simulink model "PIL"  (R2021b)
settings: Solver=FixedStepAuto  StartTime=0.0  StopTime=Inf  RelTol=1e-3
model workspace (MAT data in the model file):
  Ts = 0.001
libraries: arduinomotorcarrierlib x4
settings Model: PacingRate=2  ExtModeTrigDuration=2  Creator=cirie  LastModifiedBy=cirie
settings DataIOCC: SaveOutput=off  SaveTime=off
settings OptimizationCC: EnhancedBackFolding=on  PassReuseOutputArgsAs=Individual arguments  ZeroExternalMemoryAtStartup=off  ZeroInternalMemoryAtStartup=off  MaxStackSize=64  OptimizeBlockOrder=speed  DifferentSizesBufferReuse=on  OptimizationCustomize=off  EfficientTunableParamExpr=on
settings DebuggingCC: ParameterTunabilityLossMsg=error
settings HardwareCC: ProdBitPerPointer=32  ProdBitPerSizeT=32  ProdBitPerPtrDiffT=32  ProdLargestAtomicInteger=Long  ProdLargestAtomicFloat=Double  ProdWordSize=32  ProdHWDeviceType=ARM Compatible->ARM Cortex
settings SFSimCC: MATLABDynamicMemAlloc=off
settings RTWCC: Description=Embedded Coder  SystemTargetFile=ert.tlc  HardwareBoard=Arduino MKR WiFi 1010  TemplateMakefile=ert_default_tmf  Toolchain=Arduino ARM
settings CodeAppCC: ForceParamTrailComments=on  IgnoreCustomStorageClasses=off  OperatorAnnotations=on  SimulinkDataObjDesc=on  SFDataObjDesc=on  InsertBlockDesc=on
settings ERTTargetCC: SupportContinuousTime=on  SupportVariableSizeSignals=on  ExtModeTransport=3  ExtModeStaticAlloc=on  ExtModeStaticAllocSize=8192  ExtModeMexFile=ext_xcp  ExtModeIntrfLevel=Level2 - Open

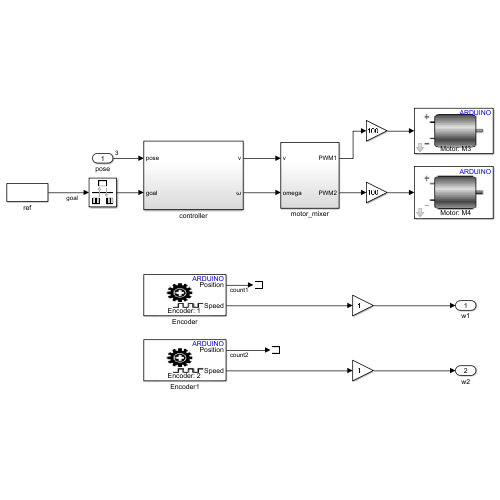
[thumbnail: Simulink's stored preview of the top-level diagram]
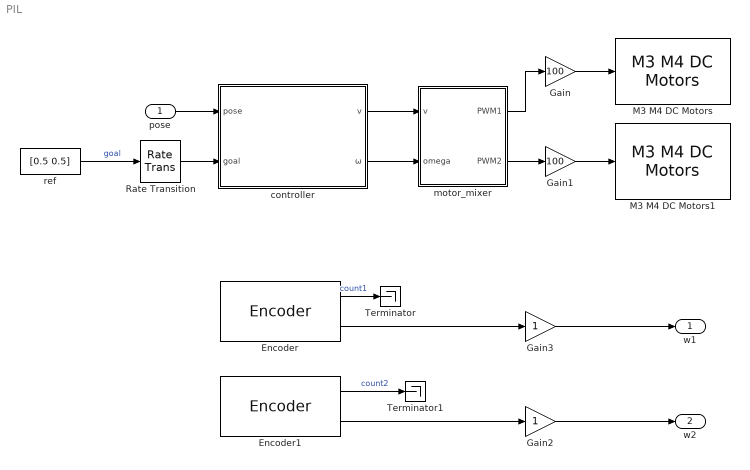
== system PIL ==
  pose : Inport  OutDataTypeStr=single  PortDimensions=3  SampleTime=[0.001,0]
  Encoder : arduinomotorcarrierlib/Encoder  SlaveAddress=uint8( hex2dec( '66' ) )  blockPlatform=ARDUINO  Encoder=1  ShowSpeed=on  ResetOption=on  SampleTime=0.01
      settings: SourceProductBaseCode=ARDUINO
  Encoder1 : arduinomotorcarrierlib/Encoder  SlaveAddress=uint8( hex2dec( '66' ) )  blockPlatform=ARDUINO  Encoder=2  ShowSpeed=on  ResetOption=on  SampleTime=0.01
      settings: SourceProductBaseCode=ARDUINO
  Gain : Gain  Gain=100
  Gain1 : Gain  Gain=100
  Gain2 : Gain
  Gain3 : Gain
  M3 M4 DC Motors : arduinomotorcarrierlib/M3 M4 DC Motors  MotorNumber=M3  forwardPinNumber=3  reversePinNumber=2
      settings: SourceProductBaseCode=ARDUINO
  M3 M4 DC Motors1 : arduinomotorcarrierlib/M3 M4 DC Motors  MotorNumber=M4  forwardPinNumber=4  reversePinNumber=5
      settings: SourceProductBaseCode=ARDUINO
  Rate Transition : RateTransition  OutPortSampleTime=Ts
  Terminator : Terminator
  Terminator1 : Terminator
  controller : Subsystem
  motor_mixer : Subsystem
  ref : Constant  Value=[0.5 0.5]  SampleTime=Ts
  w1 : Outport  OutDataTypeStr=fixdt(1,64,30)  PortDimensions=[1 1]  SampleTime=[0.01,0]
  w2 : Outport  Port=2  OutDataTypeStr=fixdt(1,64,30)  PortDimensions=[1 1]  SampleTime=[0.01,0]
  wires:
  Encoder/2 -> Gain3/1
  controller/2(ω) -> motor_mixer/2(omega)
  Gain1/1 -> M3 M4 DC Motors1/1
  motor_mixer/1(PWM1) -> Gain/1
  ref/1 -> Rate Transition/1  "goal"
  Gain/1 -> M3 M4 DC Motors/1
  controller/1(v) -> motor_mixer/1(v)
  motor_mixer/2(PWM2) -> Gain1/1
  Encoder/1 -> Terminator/1  "count1"
  Encoder1/2 -> Gain2/1
  Encoder1/1 -> Terminator1/1  "count2"
  Gain3/1 -> w1/1
  Gain2/1 -> w2/1
  pose/1 -> controller/1(pose)
  Rate Transition/1 -> controller/2(goal)

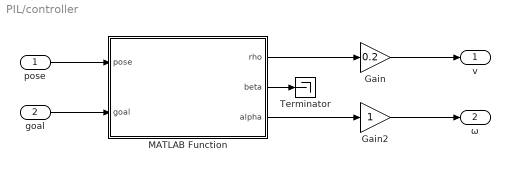
== system PIL/controller ==
  pose : Inport
  goal : Inport  Port=2
  Gain : Gain  Gain=0.2
  Gain2 : Gain
  MATLAB Function : MATLAB Function  TreatAsAtomicUnit=on
  Terminator : Terminator
  v : Outport
  ω : Outport  Port=2
  wires:
  MATLAB Function/2(beta) -> Terminator/1
  MATLAB Function/3(alpha) -> Gain2/1
  Gain2/1 -> ω/1
  Gain/1 -> v/1
  MATLAB Function/1(rho) -> Gain/1
  goal/1 -> MATLAB Function/2(goal)
  pose/1 -> MATLAB Function/1(pose)

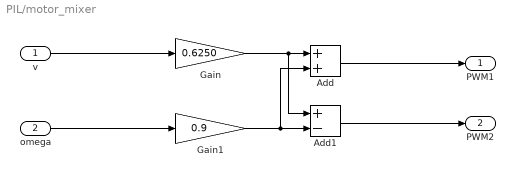
== system PIL/motor_mixer ==
  v : Inport
  omega : Inport  Port=2
  Add : Sum
  Add1 : Sum  Inputs=+-
  Gain : Gain  Gain=0.6250
  Gain1 : Gain  Gain=0.9
  PWM1 : Outport
  PWM2 : Outport  Port=2
  wires:
  v/1 -> Gain/1
  Add1/1 -> PWM2/1
  Add/1 -> PWM1/1
  Gain/1 -> Add/1, Add1/1
  Gain1/1 -> Add1/2, Add/2
  omega/1 -> Gain1/1

== matlab function PIL/controller/MATLAB Function ==
  data: pose input; rho output; goal input; beta output; alpha output
function [rho, beta, alpha] = cartesian2polar(pose, goal)

x = pose(1);
y = pose(2);
theta = pose(3);

xr = goal(1);
yr = goal(2);

dx = x-xr;
dy = y-yr;

rho = sqrt(dx^2 + dy^2);
beta = atan2(dy, dx);
alpha = beta - theta - pi;
